simulink model "sampleModel2036"  (R2023a)
settings: Solver=VariableStepAuto  StartTime=0.0  StopTime=10.0  RelTol=1e-3
libraries: hdlsllib x5, simulink x1
settings Model: Creator=user1  LastModifiedBy=user1

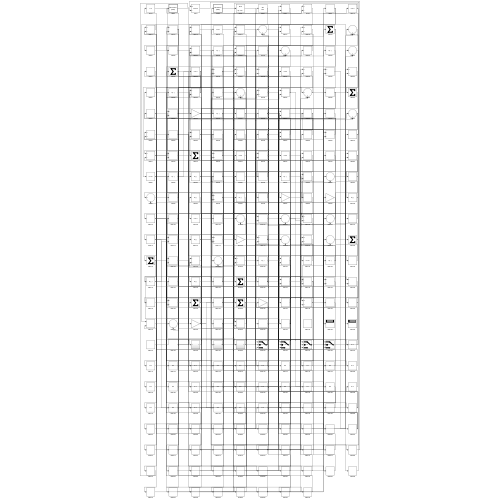
[thumbnail: Simulink's stored preview of the top-level diagram]
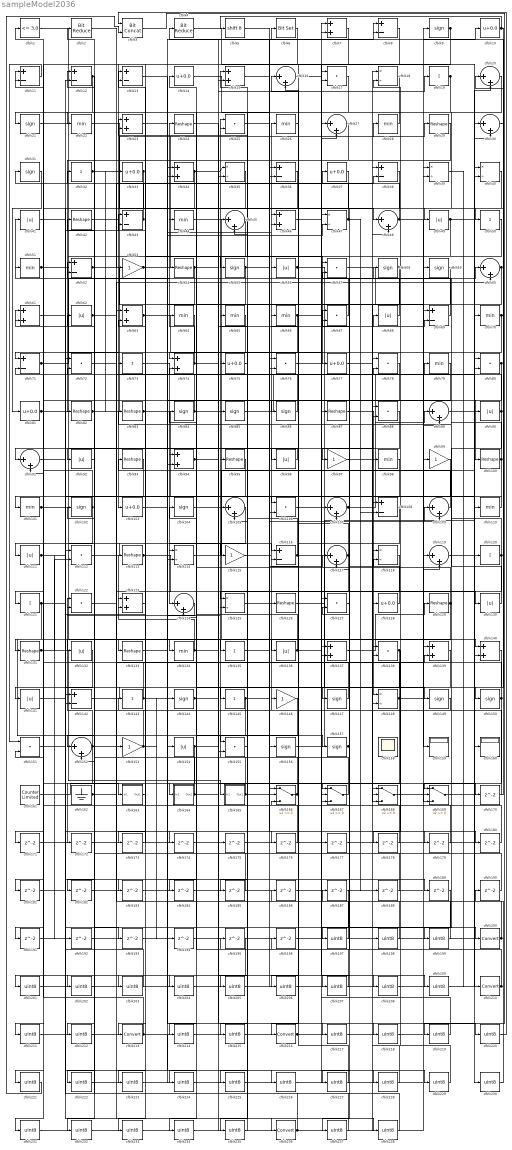
== system sampleModel2036 ==
  cfblk1 : hdlsllib/Logic and Bit Operations/Compare To Constant  relop=<=  const=3.0  OutDataTypeStr=boolean
  cfblk{10,14,33,37,75,77,81,103,128} (9 alike) : Bias  Bias=0.0  SaturateOnIntegerOverflow=off
  cfblk{24,29,42,54,82..83,87,93,95,100,113,126,129,131,133} (15 alike) : Reshape
  cfblk{22,26,28,44,51,64..66,70,79,98,101,110,134} (14 alike) : MinMax
  cfblk{9,21,31,55,58..59,84..86,102,104,144,147,149..150,156..157} (17 alike) : Signum
  cfblk{16,20,27,30,45,48,60,89,91,105,107,109,117,119,124,152} (16 alike) : Sum  Inputs=|++
  cfblk{17,25,57,67,72,76,78,80,88,106,112,122,127,138,151,155} (16 alike) : DotProduct  OutDataTypeStr=Inherit: Inherit via internal rule
  cfblk{8,11..13,36,38,43,52,69,71,108,116,142} (13 alike) : Sum  Inputs=+-
  cfblk{41,49,56,62,68,90,92,96,111,130,132,136,141,154} (14 alike) : Abs  SaturateOnIntegerOverflow=off
  cfblk{18,35,39..40,47,114,118,125,148} (9 alike) : Product  Inputs=*/  RndMeth=Zero  SaturateOnIntegerOverflow=on
  cfblk{53,97,99,115,146,153} (6 alike) : Gain
  cfblk{19,32,50,73,120..121,135,143,145} (9 alike) : Sum  Inputs=+
  cfblk{7,15,23,34,46,61,63,74,94,123,137,139..140} (13 alike) : Sum
  cfblk158 : Scope
      settings: Floating=on
  cfblk159 : Display
  cfblk160 : Display
  cfblk161 : hdlsllib/Sources/Counter Limited  uplimit=7  tsamp=-1
  cfblk162 : Ground
  cfblk163 : Subsystem
      settings: LibrarySourceBlock=|
      | hdlsllib/Ports &
      | Subsystems/Subsystem
  cfblk164 : Subsystem
      settings: LibrarySourceBlock=|
      | hdlsllib/Ports &
      | Subsystems/Subsystem
  cfblk165 : Subsystem
      settings: LibrarySourceBlock=|
      | hdlsllib/Ports &
      | Subsystems/Subsystem
  cfblk{166..169} (4 alike) : Switch  SaturateOnIntegerOverflow=off  InputSameDT=off
  cfblk{170..196} (27 alike) : Delay  SampleTime=1
  cfblk{197..199,201..209,211..212,214..215,217..235,237..238} (37 alike) : DataTypeConversion  OutDataTypeStr=uint8  SaturateOnIntegerOverflow=off  RndMeth=Floor
  cfblk2 : hdlsllib/Logic and Bit Operations/Bit Reduce  mode=AND
  cfblk{200,210,213,216,236} (5 alike) : DataTypeConversion  SaturateOnIntegerOverflow=off  RndMeth=Floor
  cfblk3 : hdlsllib/Logic and Bit Operations/Bit Concat  numInputs=2
  cfblk4 : hdlsllib/Logic and Bit Operations/Bit Reduce  mode=AND
  cfblk5 : ArithShift  BitShiftNumber=8
  cfblk6 : simulink/Logic and Bit Operations/Bit Set  iBit=0
      settings: LibrarySourceBlock=|
      | hdlsllib/Logic and Bit
      | Operations/Bit Set
  wires:
  cfblk149/1 -> cfblk26/1
  cfblk65/1 -> cfblk71/1
  cfblk72/1 -> cfblk236/1
  cfblk80/1 -> cfblk100/1, cfblk140/2
  cfblk82/1 -> cfblk28/1, cfblk33/1
  cfblk167/1 -> cfblk25/1
  cfblk28/1 -> cfblk21/1
  cfblk81/1 -> cfblk135/1, cfblk147/1
  cfblk75/1 -> cfblk155/1
  cfblk31/1 -> cfblk81/1
  cfblk169/1 -> cfblk4/1
  cfblk69/1 -> cfblk41/1
  cfblk142/1 -> cfblk145/1
  cfblk161/1 -> cfblk163/1(In1)
  cfblk9/1 -> cfblk103/1, cfblk67/2
  cfblk153/1 -> cfblk144/1, cfblk102/1, cfblk123/1, cfblk194/1
  cfblk14/1 -> cfblk126/1
  cfblk110/1 -> cfblk101/1
  cfblk115/1 -> cfblk46/1
  cfblk43/1 -> cfblk31/1, cfblk32/1
  cfblk120/1 -> cfblk148/1, cfblk51/1
  cfblk116/1 -> cfblk23/1, cfblk138/2
  cfblk107/1 -> cfblk70/1, cfblk108/2
  cfblk56/1 -> cfblk149/1, cfblk138/1
  cfblk18/1 -> cfblk216/1
  cfblk68/1 -> cfblk56/1
  cfblk53/1 -> cfblk29/1, cfblk8/2
  cfblk168/1 -> cfblk59/1
  cfblk67/1 -> cfblk24/1
  cfblk1/1 -> cfblk97/1
  cfblk128/1 -> cfblk93/1
  cfblk34/1 -> cfblk35/1, cfblk232/1
  cfblk156/1 -> cfblk109/1
  cfblk144/1 -> cfblk68/1, cfblk19/1
  cfblk70/1 -> cfblk20/1, cfblk114/2
  cfblk154/1 -> cfblk6/1, cfblk212/1
  cfblk147/1 -> cfblk11/1
  cfblk85/1 -> cfblk78/2
  cfblk15/1 -> cfblk36/1
  cfblk152/1 -> cfblk122/1, cfblk139/2, cfblk172/1
  cfblk137/1 -> cfblk129/1
  cfblk84/1 -> cfblk168/1, cfblk114/1, cfblk13/2
  cfblk57/1 -> cfblk159/1
  cfblk20/1 -> cfblk49/1
  cfblk11/1 -> cfblk151/1
  cfblk97/1 -> cfblk89/1
  cfblk166/1 -> cfblk95/1, cfblk105/2
  cfblk90/1 -> cfblk71/2, cfblk199/1
  cfblk130/1 -> cfblk83/1
  cfblk123/1 -> cfblk43/1
  cfblk101/1 -> cfblk116/1, cfblk148/2, cfblk238/1
  cfblk126/1 -> cfblk80/2
  cfblk121/1 -> cfblk165/1(In1), cfblk123/2
  cfblk73/1 -> cfblk124/1
  cfblk35/1 -> cfblk164/1(In1)
  cfblk124/1 -> cfblk122/2
  cfblk58/1 -> cfblk125/1, cfblk225/1
  cfblk86/1 -> cfblk15/1
  cfblk102/1 -> cfblk61/1, cfblk111/1
  cfblk29/1 -> cfblk82/1
  cfblk113/1 -> cfblk156/1, cfblk47/2
  cfblk125/1 -> cfblk8/1
  cfblk51/1 -> cfblk73/1, cfblk191/1
  cfblk44/1 -> cfblk128/1
  cfblk87/1 -> cfblk98/1
  cfblk83/1 -> cfblk154/1, cfblk160/1
  cfblk104/1 -> cfblk15/2
  cfblk37/1 -> cfblk92/1
  cfblk30/1 -> cfblk150/1
  cfblk59/1 -> cfblk167/1
  cfblk7/1 -> cfblk213/1
  cfblk114/1 -> cfblk30/1
  cfblk2/1 -> cfblk153/1
  cfblk55/1 -> cfblk140/1, cfblk94/1
  cfblk131/1 -> cfblk157/1, cfblk112/2
  cfblk100/1 -> cfblk52/1, cfblk237/1
  cfblk77/1 -> cfblk90/1
  cfblk47/1 -> cfblk25/2, cfblk188/1
  cfblk143/1 -> cfblk125/2, cfblk62/1
  cfblk76/1 -> cfblk200/1
  cfblk4/1 -> cfblk120/1
  cfblk88/1 -> cfblk137/2
  cfblk136/1 -> cfblk104/1, cfblk60/1
  cfblk108/1 -> cfblk136/1
  cfblk89/1 -> cfblk110/1
  cfblk103/1 -> cfblk46/2
  cfblk96/1 -> cfblk91/1
  cfblk117/1 -> cfblk66/1, cfblk235/1
  cfblk32/1 -> cfblk132/1, cfblk189/1
  cfblk112/1 -> cfblk115/1
  cfblk155/1 -> cfblk65/1
  cfblk79/1 -> cfblk131/1
  cfblk145/1 -> cfblk168/2, cfblk184/1
  cfblk71/1 -> cfblk44/1, cfblk183/1
  cfblk135/1 -> cfblk117/1
  cfblk6/1 -> cfblk141/1
  cfblk163/1(Out1) -> cfblk143/1
  cfblk52/1 -> cfblk139/1, cfblk37/1
  cfblk10/1 -> cfblk5/1, cfblk50/1
  cfblk60/1 -> cfblk166/2, cfblk167/3
  cfblk61/1 -> cfblk142/1
  cfblk62/1 -> cfblk130/1, cfblk134/1
  cfblk134/1 -> cfblk113/1, cfblk217/1
  cfblk148/1 -> cfblk10/1, cfblk42/1, cfblk181/1
  cfblk54/1 -> cfblk94/2, cfblk179/1
  cfblk19/1 -> cfblk74/1, cfblk55/1
  cfblk92/1 -> cfblk12/1
  cfblk36/1 -> cfblk152/1
  cfblk22/1 -> cfblk48/1
  cfblk50/1 -> cfblk106/1
  cfblk38/1 -> cfblk142/2
  cfblk42/1 -> cfblk53/1
  cfblk129/1 -> cfblk84/1, cfblk75/1, cfblk201/1
  cfblk25/1 -> cfblk109/2
  cfblk164/1(Out1) -> cfblk13/1, cfblk169/2
  cfblk74/1 -> cfblk54/1, cfblk169/3
  cfblk21/1 -> cfblk77/1
  cfblk138/1 -> cfblk167/2, cfblk178/1
  cfblk8/1 -> cfblk86/1
  cfblk63/1 -> cfblk107/2, cfblk218/1
  cfblk150/1 -> cfblk169/1, cfblk58/1
  cfblk165/1(Out1) -> cfblk38/2, cfblk61/2
  cfblk12/1 -> cfblk152/2, cfblk22/1
  cfblk66/1 -> cfblk168/3, cfblk185/1
  cfblk17/1 -> cfblk96/1
  cfblk48/1 -> cfblk69/1, cfblk2/1
  cfblk94/1 -> cfblk106/2, cfblk124/2
  cfblk141/1 -> cfblk43/2
  cfblk109/1 -> cfblk16/2
  cfblk39/1 -> cfblk210/1
  cfblk23/1 -> cfblk88/2
  cfblk46/1 -> cfblk87/1
  cfblk91/1 -> cfblk108/1
  cfblk157/1 -> cfblk67/1, cfblk117/2
  cfblk133/1 -> cfblk34/1
  cfblk111/1 -> cfblk11/2, cfblk192/1, cfblk193/1, cfblk229/1
  cfblk33/1 -> cfblk121/1, cfblk231/1
  cfblk49/1 -> cfblk133/1, cfblk155/2, cfblk30/2
  cfblk106/1 -> cfblk69/2
  cfblk162/1 -> cfblk79/1, cfblk60/2
  cfblk16/1 -> cfblk170/1
  cfblk170/1 -> cfblk23/2
  cfblk78/1 -> cfblk171/1
  cfblk171/1 -> cfblk107/1
  cfblk172/1 -> cfblk36/2
  cfblk95/1 -> cfblk173/1
  cfblk173/1 -> cfblk63/2
  cfblk151/1 -> cfblk174/1
  cfblk174/1 -> cfblk105/1
  cfblk175/1 -> cfblk17/2
  cfblk41/1 -> cfblk176/1
  cfblk176/1 -> cfblk1/1
  cfblk177/1 -> cfblk80/1
  cfblk178/1 -> cfblk91/2
  cfblk179/1 -> cfblk166/3
  cfblk5/1 -> cfblk180/1
  cfblk180/1 -> cfblk116/2
  cfblk181/1 -> cfblk12/2
  cfblk93/1 -> cfblk182/1
  cfblk182/1 -> cfblk137/1
  cfblk183/1 -> cfblk89/2
  cfblk184/1 -> cfblk38/1
  cfblk185/1 -> cfblk74/2
  cfblk188/1 -> cfblk52/2
  cfblk190/1 -> cfblk166/1
  cfblk191/1 -> cfblk48/2
  cfblk192/1 -> cfblk34/2
  cfblk193/1 -> cfblk35/2
  cfblk194/1 -> cfblk20/2
  cfblk196/1 -> cfblk88/1
  cfblk127/1 -> cfblk197/1
  cfblk197/1 -> cfblk57/1
  cfblk198/1 -> cfblk127/1
  cfblk199/1 -> cfblk127/2
  cfblk200/1 -> cfblk57/2, cfblk63/1
  cfblk201/1 -> cfblk76/1
  cfblk187/1 -> cfblk202/1
  cfblk202/1 -> cfblk76/2
  cfblk99/1 -> cfblk203/1
  cfblk203/1 -> cfblk112/1
  cfblk140/1 -> cfblk204/1
  cfblk204/1 -> cfblk99/1
  cfblk146/1 -> cfblk205/1
  cfblk205/1 -> cfblk177/1
  cfblk26/1 -> cfblk206/1
  cfblk206/1 -> cfblk146/1
  cfblk40/1 -> cfblk207/1
  cfblk207/1 -> cfblk14/1
  cfblk24/1 -> cfblk208/1
  cfblk208/1 -> cfblk40/1
  cfblk186/1 -> cfblk209/1
  cfblk209/1 -> cfblk40/2
  cfblk210/1 -> cfblk187/1, cfblk186/1, cfblk47/1
  cfblk132/1 -> cfblk211/1
  cfblk211/1 -> cfblk39/1
  cfblk212/1 -> cfblk39/2
  cfblk213/1 -> cfblk151/2, cfblk226/1
  cfblk105/1 -> cfblk214/1
  cfblk214/1 -> cfblk7/1
  cfblk189/1 -> cfblk215/1
  cfblk215/1 -> cfblk7/2
  cfblk216/1 -> cfblk198/1, cfblk196/1
  cfblk217/1 -> cfblk18/1
  cfblk218/1 -> cfblk18/2
  cfblk3/1 -> cfblk219/1
  cfblk219/1 -> cfblk17/1
  cfblk13/1 -> cfblk220/1
  cfblk220/1 -> cfblk3/1
  cfblk195/1 -> cfblk221/1
  cfblk221/1 -> cfblk3/2
  cfblk64/1 -> cfblk222/1
  cfblk222/1 -> cfblk175/1
  cfblk98/1 -> cfblk223/1
  cfblk223/1 -> cfblk64/1
  cfblk27/1 -> cfblk224/1
  cfblk224/1 -> cfblk9/1
  cfblk225/1 -> cfblk27/1
  cfblk226/1 -> cfblk27/2
  cfblk118/1 -> cfblk227/1
  cfblk227/1 -> cfblk16/1
  cfblk122/1 -> cfblk228/1
  cfblk228/1 -> cfblk118/1
  cfblk229/1 -> cfblk118/2
  cfblk119/1 -> cfblk230/1
  cfblk230/1 -> cfblk190/1
  cfblk231/1 -> cfblk119/1
  cfblk232/1 -> cfblk119/2
  cfblk45/1 -> cfblk233/1
  cfblk233/1 -> cfblk85/1
  cfblk139/1 -> cfblk234/1
  cfblk234/1 -> cfblk45/1
  cfblk235/1 -> cfblk45/2
  cfblk236/1 -> cfblk195/1, cfblk78/1
  cfblk237/1 -> cfblk72/1
  cfblk238/1 -> cfblk72/2

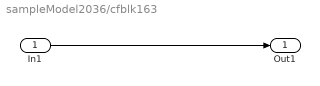
== system sampleModel2036/cfblk163 ==
  In1 : Inport
  Out1 : Outport
  wires:
  In1/1 -> Out1/1

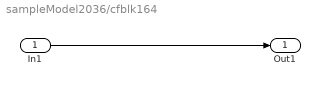
== system sampleModel2036/cfblk164 ==
  In1 : Inport
  Out1 : Outport
  wires:
  In1/1 -> Out1/1

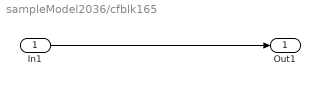
== system sampleModel2036/cfblk165 ==
  In1 : Inport
  Out1 : Outport
  wires:
  In1/1 -> Out1/1
